simulink model "T3_A_Simulink"  (R2024b)
settings: Solver=VariableStepAuto  StartTime=0.0  StopTime=10.0  RelTol=1e-3
values from neighbouring files (symbols this model uses):
  a = [1, 5.5, 8.5, 3]    [T1_B_T3_A.m]    (also in T2_B_T3_C.m = 0.5)
  p = [0, 0, 0]    [T1_B_T3_A.m]    (also in T2_A_T3_B.m = [0, 0]; T2_B_T3_C.m = [0, 1])
settings Model: Creator=lukiq  LastModifiedBy=lukiq

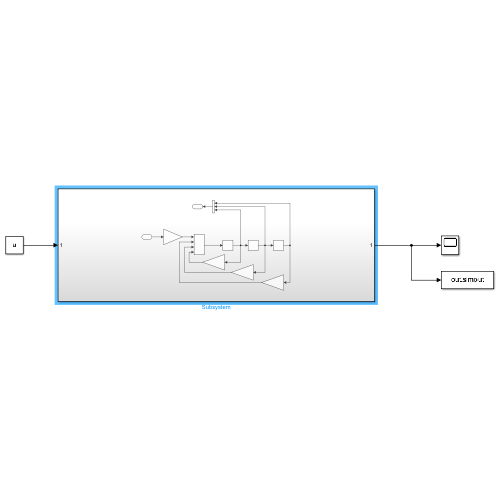
[thumbnail: Simulink's stored preview of the top-level diagram]
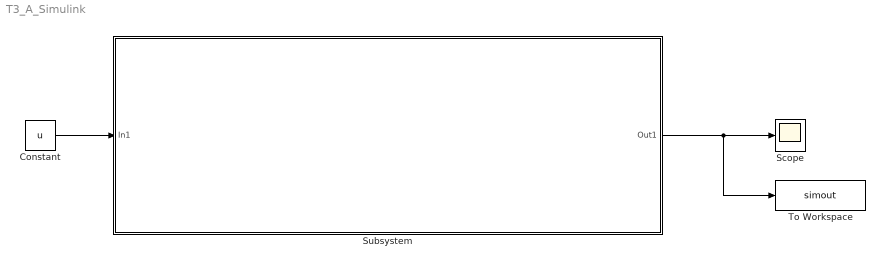
== system T3_A_Simulink ==
  Constant : Constant  Value=u
  Scope : Scope
  Subsystem : Subsystem
  To Workspace : ToWorkspace  VariableName=simout  SaveFormat=Timeseries  SampleTime=-1
  wires:
  Constant/1 -> Subsystem/1(In1)
  Subsystem/1(Out1) -> To Workspace/1, Scope/1

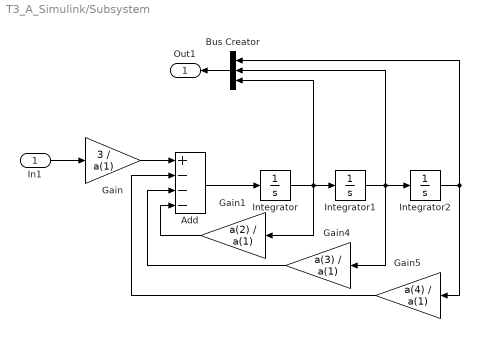
== system T3_A_Simulink/Subsystem ==
  In1 : Inport
  Add : Sum  Inputs=+---
  Bus Creator : BusCreator  Inputs=3
  Gain : Gain  Gain=3 / a(1)
  Gain1 : Gain  Gain=a(2) / a(1)
  Gain4 : Gain  Gain=a(3) / a(1)
  Gain5 : Gain  Gain=a(4) / a(1)
  Integrator : Integrator  InitialCondition=p(3)
  Integrator1 : Integrator  InitialCondition=p(2)
  Integrator2 : Integrator  InitialCondition=p(1)
  Out1 : Outport
  wires:
  In1/1 -> Gain/1
  Integrator/1 -> Bus Creator/3, Gain1/1, Integrator1/1
  Add/1 -> Integrator/1
  Gain/1 -> Add/1
  Integrator2/1 -> Bus Creator/1, Gain5/1
  Integrator1/1 -> Bus Creator/2, Integrator2/1, Gain4/1
  Gain1/1 -> Add/4
  Gain5/1 -> Add/2
  Gain4/1 -> Add/3
  Bus Creator/1 -> Out1/1
